simulink model "harnessOpenLoop2"  (R2025b)
settings: Solver=VariableStepAuto  StartTime=0.0  StopTime=600  RelTol=1e-3  AbsTol=1e-3
PreLoadFcn:
  | load DowthermProps.mat
  | load TolueneProps.mat
  | load parameters.mat
undefined symbols (not defined in the file): DOWTHERM_A, NominalStates
libraries: fl_lib x52, nesl_utility x14, SimscapeFluids_lib x6
(part 1 of 2)
settings Model: Creator=ytang  LastModifiedBy=ytang
settings SolverCC: AutoScaleAbsTol=off  AlgebraicLoopSolver=TrustRegion  MaxZcPerStep=1.0
settings DebuggingCC: UnconnectedInputMsg=warning  UnconnectedOutputMsg=warning  UnconnectedLineMsg=warning  SymbolicDimsDataTypeCodeGenerationDiagnostic=none
settings ModelReferenceCC: EnableRefExpFcnMdlSchedulingChecks=on
settings SFSimCC: CustomCodeUndefinedFunction=UseInterfaceOnly
settings RTWCC: GPUComputeCapability=3.5  DLArmComputeVersion=19.05
settings SimscapeCC: SimscapeLogType=all  SimscapeLogSimulationStatistics=on  SimscapeLogDataHistory=10000.0

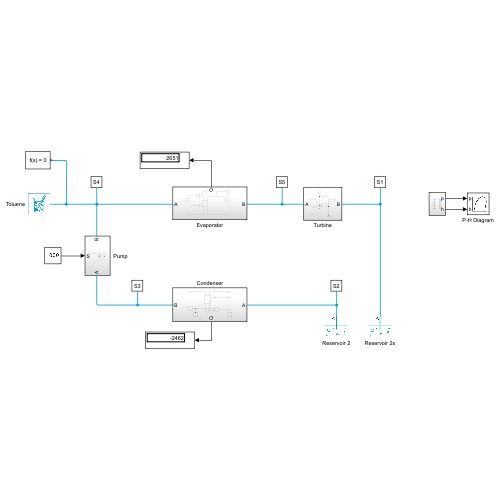
[thumbnail: Simulink's stored preview of the top-level diagram]
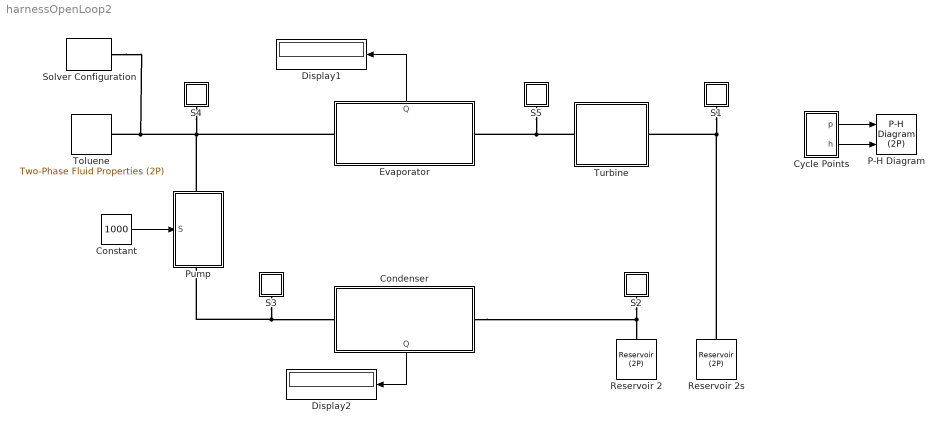
== system harnessOpenLoop2 ==
  Condenser : Subsystem
      settings: PortSchema="{\"entries\":[{\"content\":{\"sides\":[{\"content\":{\"connectorIds\":[\"LConn1\"]},\"type\":\"ConnectorPlacement.EquallySpacedRectSide\",\"uuid\":\"5f0c218a-0034-4896-a5ad-777cf4b77127\"},{\"content\":{\"connectorIds\":[\"RConn1\"],\"side\":\"RIGHT\"},\"type\":\"ConnectorPlacement.EquallySpacedRectSide\",\"uuid\":\"48348978-6e80-4dd2-96bc-6b6e5506de63\"},{\"content\":{\"side\":\"TOP\"},\"type\":\"ConnectorPlacement.EquallySpacedRectSide\",\"uuid\":\"323fdf21-ad06-4626-bb14-e50b2c3800bf\"},{\"content\":{\"connectorIds\":[\"Out1\"],\"side\":\"BOTTOM\"},\"type\":\"ConnectorPlacement.EquallySpacedRectSide\",\"uuid\":\"aca4f6cd-429e-409c-a520-3edf08891ff6\"}]},\"type\":\"ConnectorPlacement.EquallySpacedConnector\",\"uuid\":\"164d264d-504f-434e-a862-7f13511d2ab2\"}],\"packageUris\":[\"http://schema.mathworks.com/mf0/Connector/R2020b\"],\"version\":\"1.0\"}"
  Constant : Constant  Value=1000
  Cycle Points : Subsystem
  Display1 : Display
  Display2 : Display
  Evaporator : Subsystem
      settings: PortSchema="{\"entries\":[{\"content\":{\"sides\":[{\"content\":{\"connectorIds\":[\"LConn1\"]},\"type\":\"ConnectorPlacement.EquallySpacedRectSide\",\"uuid\":\"203ff6bd-d0a3-4ae0-8936-cc55cdbd18f3\"},{\"content\":{\"connectorIds\":[\"RConn1\"],\"side\":\"RIGHT\"},\"type\":\"ConnectorPlacement.EquallySpacedRectSide\",\"uuid\":\"d7ec114f-7f7a-465c-9e8c-44310e9996a8\"},{\"content\":{\"connectorIds\":[\"Out1\"],\"side\":\"TOP\"},\"type\":\"ConnectorPlacement.EquallySpacedRectSide\",\"uuid\":\"8a02f4d6-fd47-469c-93dc-df70d5198f34\"}]},\"type\":\"ConnectorPlacement.EquallySpacedConnector\",\"uuid\":\"0d570563-7e47-4bed-99ef-c8562ff711da\"}],\"packageUris\":[\"http://schema.mathworks.com/mf0/Connector/R2020b\"],\"version\":\"1.0\"}"
  P-H Diagram : SimscapeFluids_lib/Two-Phase Fluid/Utilities/P-H Diagram (2P)  p_unit=MPa  h_unit=kJ/kg
  Pump : Subsystem
      settings: PortSchema="{\"entries\":[{\"content\":{\"sides\":[{\"content\":{\"connectorIds\":[\"In1\"]},\"type\":\"ConnectorPlacement.EquallySpacedRectSide\",\"uuid\":\"bd46a3b8-4e65-4bae-b788-140c87bc05c7\"},{\"content\":{\"side\":\"RIGHT\"},\"type\":\"ConnectorPlacement.EquallySpacedRectSide\",\"uuid\":\"def7fa73-7e7d-4df6-a4d3-5611c09c4867\"},{\"content\":{\"connectorIds\":[\"LConn1\"],\"side\":\"TOP\"},\"type\":\"ConnectorPlacement.EquallySpacedRectSide\",\"uuid\":\"58b0f85b-d673-482e-aa82-3f2e724cb1a3\"},{\"content\":{\"connectorIds\":[\"RConn1\"],\"side\":\"BOTTOM\"},\"type\":\"ConnectorPlacement.EquallySpacedRectSide\",\"uuid\":\"1f6d7ee3-0842-4a9d-bce3-eda34043cffb\"}]},\"type\":\"ConnectorPlacement.EquallySpacedConnector\",\"uuid\":\"d8a4bb42-4f82-479c-8b4b-df8f3b783e33\"}],\"packageUris\":[\"http://schema.mathworks.com/mf0/Connector/R2020b\"],\"version\":\"1.0\"}"
  Reservoir 2 : fl_lib/Two-Phase Fluid/Elements/Reservoir (2P)  pressure_spec=foundation.enum.ReservoirPressureSpec2P.Specified  reservoir_pressure=NominalStates.P(2) MPa  reservoir_condensing_temperature=373.15 K  reservoir_evaporating_temperature=373.15 K  energy_spec=foundation.enum.ReservoirEnergySpec2P.Temperature  reservoir_temperature=NominalStates.T(2) degC  reservoir_quality=0.5  reservoir_void_fraction=0.5  reservoir_enthalpy=1500 kJ/kg  reservoir_internal_energy=1500 kJ/kg  reservoir_subcooling=5 deltaK  reservoir_superheating=5 deltaK  area_A=0.01 m^2
  Reservoir 2s : fl_lib/Two-Phase Fluid/Elements/Reservoir (2P)  pressure_spec=foundation.enum.ReservoirPressureSpec2P.Specified  reservoir_pressure=NominalStates.P(2) MPa  reservoir_condensing_temperature=373.15 K  reservoir_evaporating_temperature=373.15 K  energy_spec=foundation.enum.ReservoirEnergySpec2P.Temperature  reservoir_temperature=NominalStates.T(2) degC  reservoir_quality=0.5  reservoir_void_fraction=0.5  reservoir_enthalpy=1500 kJ/kg  reservoir_internal_energy=1500 kJ/kg  reservoir_subcooling=5 deltaK  reservoir_superheating=5 deltaK  area_A=0.01 m^2
  S1 : Subsystem
      mask Display: disp(get_param(gcb, 'Name'))
  S2 : Subsystem
      mask Display: disp(get_param(gcb, 'Name'))
  S3 : Subsystem
      mask Display: disp(get_param(gcb, 'Name'))
  S4 : Subsystem
      mask Display: disp(get_param(gcb, 'Name'))
  S5 : Subsystem
      mask Display: disp(get_param(gcb, 'Name'))
  Solver Configuration : nesl_utility/Solver Configuration  PhysicalDomain=network_engine_domain  SubClassName=solver  LeftPortType=input  RightPortType=generic  Tones=[]  Harmonics=[]  SimulateNoise=off  Profile=off  UseLocalSampling=off  EnableSwitchedLinearOptims=on  FrequencyDomain=off  UseCCode=off  RelTol=0.001  AbsTol=0.001  MinStep=1e-09  ToWorkspace=off  RevertToSquareIcSolve=off  NumHomotopyIterations=100  PhasorMode=off  PhasorModeNumHarmonics=1  ConsistencySolver=NEWTON_XTOL_AFTER_FTOL  IndexReductionMethod=DerivativeReplacement  DoDC=off  ResidualTolerance=1e-09  ConsistencyTolSource=GLOBAL  ConsistencyAbsTol=0.001  ConsistencyRelTol=0.001  ConsistencyTolFactor=0.001  UseLocalSolver=off  LocalSolverChoice=NE_BACKWARD_EULER_ADVANCER  ResolveIndetEquations=on  FunctionEvalNumThread=1  LocalSolverSampleTime=0.001  DoFixedCost=off  MaxNonlinIter=3  MaxModeIter=2  ComputeImpulses=off  ImpulseIterations=2  LinearAlgebra=auto  LinearAlgebraNumThread=0  EquationFormulation=NE_TIME_EF  DelaysMemoryBudget=1024  AutomaticFiltering=on  FilteringTimeConstant=0.001  PartitionStorageMethod=AS_NEEDED  PartitionMemoryBudget=1024  PartitionMethod=ROBUST  MultibodyUseLocalSolver=off  MultibodyLocalSolverChoice=ODE1  MultibodyLocalSolverSampleTime=0.001
  Toluene : fl_lib/Two-Phase Fluid/Utilities/Two-Phase Fluid Properties (2P)  u_min=Toluene.u_min kJ/kg  u_max=Toluene.u_max kJ/kg  p_TLU=Toluene.p MPa  p_crit=Toluene.p_crit MPa  critical_region=foundation.enum.critical_region.clip  p_crit_fraction=0.12  p_atm=0.101325 MPa  properties_range_check=simscape.enum.assert.action.error  q_rev=0.01 Pa  unorm_liq=Toluene.liquid.unorm  v_liq=Toluene.liquid.v m^3/kg  s_liq=Toluene.liquid.s kJ/(kg*K)  T_liq=Toluene.liquid.T K  nu_liq=Toluene.liquid.nu mm^2/s  k_liq=Toluene.liquid.k W/(m*K)  Pr_liq=Toluene.liquid.Pr  u_sat_liq=Toluene.liquid.u_sat kJ/kg  unorm_vap=Toluene.vapor.unorm  v_vap=Toluene.vapor.v m^3/kg  s_vap=Toluene.vapor.s kJ/(kg*K)  T_vap=Toluene.vapor.T K  nu_vap=Toluene.vapor.nu mm^2/s  k_vap=Toluene.vapor.k W/(m*K)  Pr_vap=Toluene.vapor.Pr  u_sat_vap=Toluene.vapor.u_sat kJ/kg
      settings: InternalSimscapePortConfiguration="{\"Bottom\":[],\"Left\":[],\"Right\":[{\"id\":\"A\",\"label\":\"\",\"type\":\"foundation.two_phase_fluid.two_phase_fluid\"}],\"Top\":[]}"
  Turbine : Subsystem
  wires:
  Cycle Points/2(h) -> P-H Diagram/2
  Cycle Points/1(p) -> P-H Diagram/1
  Constant/1 -> Pump/1(S)
  Evaporator/1(Q) -> Display1/1
  Condenser/1(Q) -> Display2/1
  connections:
  Turbine/LConn1 -- S5/LConn1 -- Evaporator/RConn1
  S2/LConn1 -- Condenser/RConn1 -- Reservoir 2/LConn1
  S3/LConn1 -- Pump/RConn1 -- Condenser/LConn1
  Pump/LConn1 -- S4/LConn1 -- Evaporator/LConn1 -- Solver Configuration/RConn1 -- Toluene/RConn1
  Reservoir 2s/LConn1 -- S1/LConn1 -- Turbine/RConn1

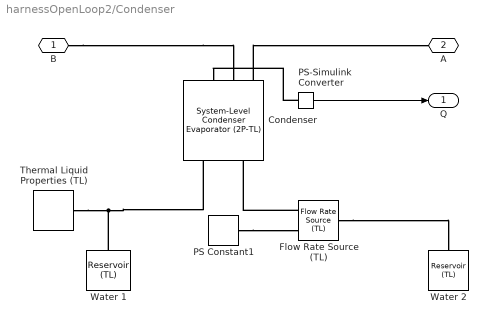
== system harnessOpenLoop2/Condenser ==
  Condenser : SimscapeFluids_lib/Heat Exchangers/Two-Phase Fluid - Thermal Liquid/System-Level Condenser Evaporator (2P-TL)  flow_arrangement=fluids.heat_exchangers.enum.SystemLevelFlowArrangement2PTL.Counter  wall_thermal_mass=false  mass_wall=1 kg  cp_wall=490 J/(K*kg)  nominal_init_wall=true  T_wall_init=293.15 K  area_A1=0.01 m^2  area_B1=0.01 m^2  area_A2=0.01 m^2  area_B2=0.01 m^2  operating_condition_2P=fluids.heat_exchangers.enum.SystemLevelOperatingCondition2PTL.Condenser  mdot_nominal_2P=Condenser.Fluid.mdot kg/s  delta_p_nominal_2P=0.0001 MPa  pressure_spec_cond_2P=fluids.heat_exchangers.enum.SystemLevelPressureSpecCondenser2P.InletPressure  pressure_spec_evap_2P=fluids.heat_exchangers.enum.SystemLevelPressureSpecEvaporator2P.InletPressure  p_in_nominal_2P=NominalStates.P(2) MPa  T_cond_nominal_2P=313.15 K  T_evap_nominal_2P=243.15 K  inlet_spec_2P=fluids.heat_exchangers.enum.SystemLevelInletSpec2P.Temperature  T_in_nominal_2P=NominalStates.T(2) degC  h_in_nominal_2P=440 kJ/kg  x_in_nominal_2P=1  capacity_spec_2P=fluids.heat_exchangers.enum.SystemLevelCapacitySpec.HeatTransfer  Q_nominal=Condenser.Heat kW  outlet_spec_cond_2P=fluids.heat_exchangers.enum.SystemLevelOutletSpecCondenser2P.Enthalpy  outlet_spec_evap_2P=fluids.heat_exchangers.enum.SystemLevelOutletSpecEvaporator2P.Enthalpy  delta_T_sub_nominal_2P=5 deltaK  delta_T_sup_nominal_2P=5 deltaK  h_out_nominal_2P=250 kJ/kg  x_out_nominal_2P=0  volume_2P=0.2 m^3  nominal_init_2P=true  energy_spec_2P=foundation.enum.energy_spec.enthalpy  p_init_2P=0.101325 MPa  T_init_2P=293.15 K  x_init_2P=0.5  alpha_init_2P=0.5  h_init_2P=1500 kJ/kg  u_init_2P=1500 kJ/kg  mdot_nominal_TL=Condenser.Water.mdot kg/s  delta_p_nominal_TL=0.0001 MPa  p_in_nominal_TL=0.101325 MPa  T_in_nominal_TL=Condenser.Water.Tin degC  volume_TL=0.2 m^3  nominal_init_TL=true  p_init_TL=0.101325 MPa  T_init_TL=293.15 K  a_liq_2P=0.023  a_mix_2P=0.005  a_vap_2P=0.023  b_2P=0.8  c_2P=0.33  a_TL=0.023  b_TL=0.8  c_TL=0.33
      settings: InternalSimscapePortConfiguration="{\"Bottom\":[],\"Left\":[{\"id\":\"A1\",\"label\":\"A1\",\"type\":\"foundation.two_phase_fluid.two_phase_fluid\"},{\"id\":\"B1\",\"label\":\"B1\",\"type\":\"foundation.two_phase_fluid.two_phase_fluid\"}],\"Right\":[{\"id\":\"A2\",\"label\":\"A2\",\"type\":\"foundation.thermal_liquid.thermal_liquid\"},{\"id\":\"B2\",\"label\":\"B2\",\"type\":\"foundation.thermal_liquid.thermal_liquid\"}],\"Top\":[{\"id\":\"Q1\",\"label\":\"Q1\",\"type\":\"output\"},{\"id\":\"Q2\",\"label\":\"Q2\",\"type\":\"output\"}]}"
  Flow Rate Source (TL) : fl_lib/Thermal Liquid/Sources/Flow Rate Source (TL)  source_type=foundation.enum.constant_controlled.controlled  flow_type=foundation.enum.mass_volumetric_flow.mass  mass_flow=0 kg/s  volumetric_flow=0 m^3/s  power_spec=foundation.enum.power_spec.isentropic  area=0.01 m^2
  PS Constant1 : fl_lib/Physical Signals/Sources/PS Constant  constant=Condenser.Water.mdot kg/s
  PS-Simulink Converter : nesl_utility/PS-Simulink Converter  PhysicalDomain=network_engine_domain  SubClassName=ps_output  LeftPortType=input  RightPortType=output  PseudoPeriodic=off  Frequencies=[]  VectorFormat=inherit  Unit=kW  AffineConversion=off
  Thermal Liquid Properties (TL) : SimscapeFluids_lib/Thermal Liquid/Utilities/Thermal Liquid Properties (TL)  fluid_list=fluids.thermal_liquid.utilities.enum.thermal_liquid_fluid_list.water  concentration_param_EG=fluids.thermal_liquid.utilities.enum.thermal_liquid_concentration.volume_fraction  concentration_param_PG=fluids.thermal_liquid.utilities.enum.thermal_liquid_concentration.volume_fraction  c_mass_SW=3.5e-3  c_mass_EG=0.1  c_mass_PG=0.1  c_mass_GL=0.1  c_vol_EG=0.1  c_vol_PG=0.1  beta_const_EG=2.1791 GPa  beta_const_PG=2.1791 GPa  beta_const_GL=2.1791 GPa  p_min_EG=0.01 MPa  p_min_PG=0.01 MPa  p_min_GL=0.01 MPa  p_max_EG=50 MPa  p_max_PG=50 MPa  p_max_GL=50 MPa  p_atm=0.101325 MPa  properties_range_check=simscape.enum.assert.action.error
  Water 1 : fl_lib/Thermal Liquid/Elements/Reservoir (TL)  pressure_spec=foundation.enum.pressure_spec.atmospheric  reservoir_pressure=0.101325 MPa  reservoir_temperature=Condenser.Water.Tin degC  area=0.01 m^2
  Water 2 : fl_lib/Thermal Liquid/Elements/Reservoir (TL)  pressure_spec=foundation.enum.pressure_spec.atmospheric  reservoir_pressure=0.101325 MPa  reservoir_temperature=Condenser.Water.Tout degC  area=0.01 m^2
  B : PMIOPort  Side=Left
  A : PMIOPort  Port=2  Side=Right
  Q : Outport
  wires:
  PS-Simulink Converter/1 -> Q/1
  connections:
  Flow Rate Source (TL)/RConn1 -- Water 2/LConn1
  PS-Simulink Converter/LConn1 -- Condenser/LConn3
  Water 1/LConn1 -- Condenser/RConn2 -- Thermal Liquid Properties (TL)/RConn1
  Flow Rate Source (TL)/LConn1 -- Condenser/RConn1
  PS Constant1/RConn1 -- Flow Rate Source (TL)/LConn2
  B/RConn1 -- Condenser/LConn2
  Condenser/LConn1 -- A/RConn1

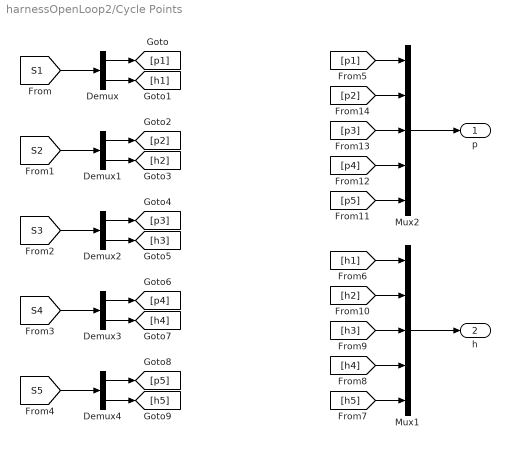
== system harnessOpenLoop2/Cycle Points ==
  Demux{,1..4} (5 alike) : Demux  Outputs=2
  Mux1 : Mux  Inputs=5
  Mux2 : Mux  Inputs=5
  p : Outport
  h : Outport  Port=2
  wires:
  Mux1/1 -> h/1
  [S1] -> Demux/1
  [S2] -> Demux1/1
  [S3] -> Demux2/1
  [S4] -> Demux3/1
  [S5] -> Demux4/1
  Mux2/1 -> p/1
  Demux/1 -> [p1]
  [p1] -> Mux2/1
  Demux2/2 -> [h3]
  [h3] -> Mux1/3
  Demux3/2 -> [h4]
  [h4] -> Mux1/4
  Demux4/2 -> [h5]
  [h5] -> Mux1/5
  Demux1/2 -> [h2]
  [h2] -> Mux1/2
  Demux/2 -> [h1]
  [h1] -> Mux1/1
  Demux3/1 -> [p4]
  [p4] -> Mux2/4
  Demux4/1 -> [p5]
  [p5] -> Mux2/5
  Demux1/1 -> [p2]
  [p2] -> Mux2/2
  Demux2/1 -> [p3]
  [p3] -> Mux2/3

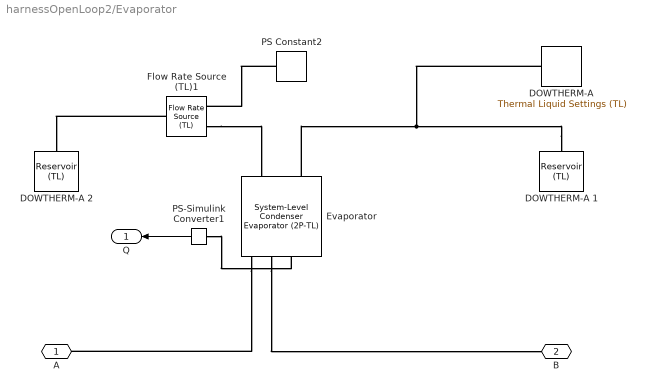
== system harnessOpenLoop2/Evaporator ==
  DOWTHERM-A : fl_lib/Thermal Liquid/Utilities/Thermal Liquid Settings (TL)  table_dimensions=foundation.enum.table_dimensions_TL.one_dimensional  T_TLU=DOWTHERM_A.T degC  p_TLU=[0.01, 0.1, 5 : 5 : 50] MPa  p_atm=0.101325 MPa  pT_region_flag=foundation.enum.pT_region_TL.min_max  T_min=273.16 K  T_max=373.16 K  p_min=0.01 MPa  p_max=50 MPa  T_min_1D=DOWTHERM_A.T(1) degC  T_max_1D=DOWTHERM_A.T(end) degC  p_min_1D=0.01 MPa  p_max_1D=50 MPa  pT_validity_TLU=[1, 1, 1, 1, 1, 1, 1, 1, 1, 1, 1, 1; 1, 1, 1, 1, 1, 1, 1, 1, 1, 1, 1, 1; 1, 1, 1, 1, 1, 1, 1, 1, 1, 1, 1, 1; 1, 1, 1, 1, 1, 1, 1, 1, 1, 1, 1, 1; 1, 1, 1, 1, 1, 1, 1, 1, 1, 1, 1, 1; 0, 1, 1, 1, 1, 1, 1, 1, 1, 1, 1, 1; 0, 1, 1, 1, 1, 1, 1, 1, 1, 1, 1, 1; 0, 1, 1, 1, 1, 1, 1, 1, 1, 1, 1, 1; 0, 1, 1, 1, 1, 1, 1, 1, 1, 1, 1, 1; 0, 1, 1, 1, 1, 1, 1, 1, 1, 1, 1, 1; 0, 0, 1, 1, 1, 1, 1, 1, 1, 1, 1, 1]  properties_range_check=simscape.enum.assert.action.error  rho_parameterization_2D=foundation.enum.rho_parameterization_2D.rho_beta_alpha  rho_parameterization_1D=foundation.enum.rho_parameterization_1D.rho_vector  rho_TLU=[999.7973, 999.8431, 1002.3216, 1004.8218, 1007.293, 1009.7358, 1012.1506, 1014.5379, 1016.8979, 1019.2311, 1021.538, 1023.8188; 999.6579, 999.7009, 1002.0303, 1004.382, 1006.7084, 1009.0101, 1011.2874, 1013.5407, 1015.7703, 1017.9766, 1020.1599, 1022.3206; 998.1632, 998.2045, 1000.4375, 1002.6924, 1004.9239, 1007.1324, 1009.3183, 1011.4819, 1013.6236, 1015.7438, 1017.8428, 1019.921; 995.6057, 995.6458, 997.8186, 1000.0128, 1002.1841, 1004.3332, 1006.4603, 1008.566, 1010.6505, 1012.7144, 1014.758, 1016.7815; 992.1724, 992.2119, 994.3513, 996.5113, 998.6484, 1000.7633, 1002.8563, 1004.928, 1006.9788, 1009.009, 1011.0192, 1013.0097; 988.02, 988.0299, 990.1568, 992.3035, 994.4268, 996.5273, 998.6056, 1000.6622, 1002.6976, 1004.7123, 1006.7067, 1008.6813; 983.18, 983.1901, 985.3217, 987.4721, 989.5983, 991.7008, 993.7803, 995.8374, 997.8726, 999.8864, 1001.8795, 1003.8522; 977.75, 977.7583, 979.9094, 982.0783, 984.2216, 986.34, 988.4343, 990.505, 992.5529, 994.5786, 996.5825, 998.5654; 971.77, 971.7836, 973.9673, 976.1678, 978.3409, 980.4876, 982.6087, 984.7049, 986.7768, 988.8254, 990.8511, 992.8545; 965.26, 965.3023, 967.5311, 969.7753, 971.9901, 974.1764, 976.3354, 978.4676, 980.5741, 982.6556, 984.7129, 986.7465; 958.62, 958.6315, 960.627, 962.9267, 965.1944, 967.4314, 969.6387, 971.8173, 973.9681, 976.0921, 978.19, 980.2628] kg/m^3  beta_TLU=[1.9649, 1.9654, 1.9929, 2.0213, 2.0499, 2.0787, 2.1078, 2.1372, 2.1668, 2.1966, 2.2268, 2.2572; 2.0913, 2.0918, 2.1191, 2.1471, 2.1752, 2.2036, 2.2322, 2.261, 2.2899, 2.3191, 2.3485, 2.3781; 2.1786, 2.1791, 2.2067, 2.235, 2.2634, 2.2919, 2.3206, 2.3494, 2.3784, 2.4075, 2.4367, 2.4661; 2.2332, 2.2337, 2.2619, 2.2908, 2.3197, 2.3487, 2.3778, 2.407, 2.4363, 2.4657, 2.4951, 2.5246; 2.26, 2.2605, 2.2895, 2.3191, 2.3487, 2.3784, 2.4081, 2.4378, 2.4675, 2.4973, 2.5272, 2.5571; 2.2638, 2.2638, 2.2936, 2.324, 2.3544, 2.3848, 2.4151, 2.4455, 2.4758, 2.5062, 2.5365, 2.5669; 2.2472, 2.2472, 2.2779, 2.3092, 2.3403, 2.3715, 2.4025, 2.4336, 2.4646, 2.4955, 2.5264, 2.5573; 2.214, 2.214, 2.2455, 2.2776, 2.3096, 2.3415, 2.3733, 2.405, 2.4367, 2.4683, 2.4998, 2.5313; 2.1668, 2.1668, 2.1992, 2.2321, 2.2649, 2.2976, 2.3301, 2.3626, 2.3949, 2.4272, 2.4593, 2.4914; 2.1081, 2.1081, 2.1413, 2.175, 2.2086, 2.2421, 2.2754, 2.3085, 2.3415, 2.3744, 2.4072, 2.4399; 2.0494, 2.0494, 2.0739, 2.1084, 2.1428, 2.177, 2.211, 2.2449, 2.2786, 2.3121, 2.3455, 2.3788] GPa  alpha_TLU=1e-4 * [-.679, -.676, -.49, -.307, -.13, .041, .206, .365, .519, .668, .811, .949; .878, .881, .998, 1.114, 1.227, 1.337, 1.445, 1.549, 1.651, 1.75, 1.846, 1.939; 2.068, 2.069, 2.141, 2.213, 2.283, 2.352, 2.42, 2.486, 2.551, 2.614, 2.676, 2.736; 3.034, 3.035, 3.074, 3.113, 3.152, 3.191, 3.229, 3.267, 3.305, 3.341, 3.377, 3.413; 3.855, 3.856, 3.87, 3.884, 3.899, 3.914, 3.93, 3.946, 3.961, 3.977, 3.993, 4.009; 4.578, 4.578, 4.572, 4.566, 4.562, 4.558, 4.555, 4.552, 4.55, 4.549, 4.548, 4.547; 5.233, 5.233, 5.209, 5.186, 5.165, 5.144, 5.125, 5.107, 5.09, 5.074, 5.059, 5.045; 5.84, 5.84, 5.801, 5.762, 5.725, 5.691, 5.657, 5.625, 5.595, 5.566, 5.538, 5.512; 6.414, 6.414, 6.36, 6.307, 6.256, 6.208, 6.161, 6.117, 6.074, 6.033, 5.994, 5.956; 6.967, 6.967, 6.898, 6.831, 6.766, 6.705, 6.646, 6.589, 6.535, 6.482, 6.432, 6.384; 7.519, 7.519, 7.423, 7.342, 7.264, 7.189, 7.118, 7.049, 6.983, 6.92, 6.859, 6.8] 1/K  rho_TLU_2=[999.7973, 999.8431, 1002.3216, 1004.8218, 1007.293, 1009.7358, 1012.1506, 1014.5379, 1016.8979, 1019.2311, 1021.538, 1023.8188; 999.6579, 999.7009, 1002.0303, 1004.382, 1006.7084, 1009.0101, 1011.2874, 1013.5407, 1015.7703, 1017.9766, 1020.1599, 1022.3206; 998.1632, 998.2045, 1000.4375, 1002.6924, 1004.9239, 1007.1324, 1009.3183, 1011.4819, 1013.6236, 1015.7438, 1017.8428, 1019.921; 995.6057, 995.6458, 997.81864, 1000.0128, 1002.1841, 1004.3332, 1006.4603, 1008.566, 1010.6505, 1012.7144, 1014.758, 1016.7815; 992.1724, 992.2119, 994.3513, 996.5113, 998.6484, 1000.7633, 1002.8563, 1004.928, 1006.9788, 1009.009, 1011.0192, 1013.0097; 988.02, 988.0299, 990.1568, 992.3035, 994.4268, 996.5273, 998.6056, 1000.6622, 1002.6976, 1004.7123, 1006.7067, 1008.6813; 983.18, 983.1901, 985.3217, 987.4721, 989.5983, 991.7008, 993.7803, 995.8374, 997.8726, 999.8864, 1001.8795, 1003.8522; 977.75, 977.7583, 979.9094, 982.0783, 984.2216, 986.34, 988.4343, 990.505, 992.5529, 994.5786, 996.5825, 998.5654; 971.77, 971.7836, 973.9673, 976.1678, 978.3409, 980.4876, 982.6087, 984.7049, 986.7768, 988.8254, 990.8511, 992.8545; 965.26, 965.3023, 967.5311, 969.7753, 971.9901, 974.1764, 976.3354, 978.4676, 980.5741, 982.6556, 984.7129, 986.7465; 958.62, 958.6315, 960.627, 962.9267, 965.1944, 967.4314, 969.6387, 971.8173, 973.9681, 976.0921, 978.19, 980.2628] kg/m^3  rho_ref_3=998.21 kg/m^3  T_ref_3=293.16 K  p_ref_3=0.101325 MPa  beta_const_3=2.1791 GPa  alpha_const_3=2.0691e-4 1/K  rho_TLU_4=DOWTHERM_A.rho kg/m^3  beta_const_4=0.5 GPa  p_ref_4=0.101325 MPa  rho_ref_5=998.21 kg/m^3  T_ref_5=293.16 K  p_ref_5=0.101325 MPa  beta_const_5=2.1791 GPa  alpha_const_5=2.0691e-4 1/K  u_parameterization_2D=foundation.enum.u_parameterization_2D.u_cp  u_parameterization_1D=foundation.enum.u_parameterization_1D.cp  u_TLU=[.0002, .0018, .086, .1588, .219, .267, .3034, .3288, .3436, .3483, .3435, .3294; 42.062, 42.06, 41.935, 41.804, 41.668, 41.527, 41.382, 41.233, 41.081, 40.924, 40.763, 40.599; 83.953, 83.948, 83.651, 83.349, 83.049, 82.749, 82.451, 82.153, 81.856, 81.56, 81.265, 80.971; 125.77, 125.76, 125.31, 124.86, 124.41, 123.97, 123.53, 123.1, 122.68, 122.25, 121.84, 121.42; 167.57, 167.56, 166.96, 166.37, 165.79, 165.21, 164.65, 164.09, 163.54, 163, 162.46, 161.94; 209.36, 209.36, 208.63, 207.9, 207.19, 206.48, 205.79, 205.11, 204.45, 203.79, 203.14, 202.5; 251.19, 251.19, 250.33, 249.47, 248.62, 247.79, 246.98, 246.18, 245.39, 244.62, 243.86, 243.12; 293.06, 293.06, 292.07, 291.07, 290.1, 289.14, 288.2, 287.28, 286.38, 285.49, 284.62, 283.77; 334.99, 334.99, 333.86, 332.73, 331.63, 330.54, 329.48, 328.44, 327.41, 326.41, 325.43, 324.46; 377, 377, 375.73, 374.46, 373.22, 372, 370.81, 369.64, 368.5, 367.38, 366.27, 365.19; 419.01, 419.01, 417.69, 416.27, 414.89, 413.54, 412.21, 410.91, 409.64, 408.4, 407.17, 405.98] kJ/kg  cp_TLU=[4.2199, 4.2194, 4.1957, 4.1726, 4.1508, 4.13, 4.1103, 4.0916, 4.0738, 4.0569, 4.0408, 4.0254; 4.1955, 4.1951, 4.1769, 4.1592, 4.1422, 4.1259, 4.1103, 4.0954, 4.0812, 4.0676, 4.0545, 4.0421; 4.1843, 4.184, 4.169, 4.1543, 4.1401, 4.1264, 4.1133, 4.1007, 4.0885, 4.0768, 4.0656, 4.0548; 4.1801, 4.1798, 4.1667, 4.1538, 4.1413, 4.1293, 4.1177, 4.1064, 4.0956, 4.0851, 4.075, 4.0653; 4.1796, 4.1794, 4.1675, 4.1558, 4.1444, 4.1334, 4.1227, 4.1123, 4.1023, 4.0926, 4.0832, 4.0741; 4.1813, 4.1813, 4.1702, 4.1592, 4.1484, 4.138, 4.1279, 4.1181, 4.1086, 4.0993, 4.0903, 4.0816; 4.185, 4.185, 4.1742, 4.1636, 4.1532, 4.1432, 4.1334, 4.1239, 4.1146, 4.1056, 4.0969, 4.0884; 4.1901, 4.1901, 4.1795, 4.169, 4.1588, 4.1489, 4.1393, 4.1299, 4.1207, 4.1118, 4.1032, 4.0947; 4.1968, 4.1968, 4.1862, 4.1757, 4.1655, 4.1555, 4.1458, 4.1364, 4.1273, 4.1183, 4.1096, 4.1012; 4.2052, 4.2052, 4.1944, 4.1837, 4.1733, 4.1632, 4.1534, 4.1438, 4.1345, 4.1255, 4.1166, 4.108; 4.2136, 4.2136, 4.2045, 4.1935, 4.1828, 4.1724, 4.1623, 4.1524, 4.1429, 4.1335, 4.1245, 4.1157] kJ/(K*kg)  u_TLU_2=[.0002, .0018, .086, .1588, .219, .267, .3034, .3288, .3436, .3483, .3435, .3294; 42.062, 42.06, 41.935, 41.804, 41.668, 41.527, 41.382, 41.233, 41.081, 40.924, 40.763, 40.599; 83.953, 83.948, 83.651, 83.349, 83.049, 82.749, 82.451, 82.153, 81.856, 81.56, 81.265, 80.971; 125.77, 125.76, 125.31, 124.86, 124.41, 123.97, 123.53, 123.1, 122.68, 122.25, 121.84, 121.42; 167.57, 167.56, 166.96, 166.37, 165.79, 165.21, 164.65, 164.09, 163.54, 163, 162.46, 161.94; 209.36, 209.36, 208.63, 207.9, 207.19, 206.48, 205.79, 205.11, 204.45, 203.79, 203.14, 202.5; 251.19, 251.19, 250.33, 249.47, 248.62, 247.79, 246.98, 246.18, 245.39, 244.62, 243.86, 243.12; 293.06, 293.06, 292.07, 291.07, 290.1, 289.14, 288.2, 287.28, 286.38, 285.49, 284.62, 283.77; 334.99, 334.99, 333.86, 332.73, 331.63, 330.54, 329.48, 328.44, 327.41, 326.41, 325.43, 324.46; 377, 377, 375.73, 374.46, 373.22, 372, 370.81, 369.64, 368.5, 367.38, 366.27, 365.19; 419.01, 419.01, 417.69, 416.27, 414.89, 413.54, 412.21, 410.91, 409.64, 408.4, 407.17, 405.98] kJ/kg  cp_TLU_3=[4.2199, 4.2194, 4.1957, 4.1726, 4.1508, 4.13, 4.1103, 4.0916, 4.0738, 4.0569, 4.0408, 4.0254; 4.1955, 4.1951, 4.1769, 4.1592, 4.1422, 4.1259, 4.1103, 4.0954, 4.0812, 4.0676, 4.0545, 4.0421; 4.1843, 4.184, 4.169, 4.1543, 4.1401, 4.1264, 4.1133, 4.1007, 4.0885, 4.0768, 4.0656, 4.0548; 4.1801, 4.1798, 4.1667, 4.1538, 4.1413, 4.1293, 4.1177, 4.1064, 4.0956, 4.0851, 4.075, 4.0653; 4.1796, 4.1794, 4.1675, 4.1558, 4.1444, 4.1334, 4.1227, 4.1123, 4.1023, 4.0926, 4.0832, 4.0741; 4.1813, 4.1813, 4.1702, 4.1592, 4.1484, 4.138, 4.1279, 4.1181, 4.1086, 4.0993, 4.0903, 4.0816; 4.185, 4.185, 4.1742, 4.1636, 4.1532, 4.1432, 4.1334, 4.1239, 4.1146, 4.1056, 4.0969, 4.0884; 4.1901, 4.1901, 4.1795, 4.169, 4.1588, 4.1489, 4.1393, 4.1299, 4.1207, 4.1118, 4.1032, 4.0947; 4.1968, 4.1968, 4.1862, 4.1757, 4.1655, 4.1555, 4.1458, 4.1364, 4.1273, 4.1183, 4.1096, 4.1012; 4.2052, 4.2052, 4.1944, 4.1837, 4.1733, 4.1632, 4.1534, 4.1438, 4.1345, 4.1255, 4.1166, 4.108; 4.2136, 4.2136, 4.2045, 4.1935, 4.1828, 4.1724, 4.1623, 4.1524, 4.1429, 4.1335, 4.1245, 4.1157] kJ/(K*kg)  u_TLU_4=[.0018; 42.06; 83.948; 125.76; 167.56; 209.36; 251.19; 293.06; 334.99; 377; 418.01] kJ/kg  cp_TLU_5=DOWTHERM_A.Cp kJ/(K*kg)  nu_TLU=[1.7917, 1.7914, 1.7763, 1.7615, 1.7473, 1.7338, 1.7208, 1.7085, 1.6967, 1.6854, 1.6747, 1.6645; 1.3061, 1.3059, 1.2986, 1.2914, 1.2845, 1.2779, 1.2716, 1.2656, 1.2598, 1.2543, 1.2491, 1.2441; 1.0032, 1.0032, .9995, .9959, .9924, .9891, .9859, .9829, .9801, .9774, .9748, .9724; .8006, .8005, .7987, .797, .7953, .7937, .7922, .7908, .7894, .7881, .787, .7859; .6577, .6577, .657, .6562, .6555, .6548, .6543, .6537, .6532, .6528, .6523, .652; .553, .553, .5529, .5527, .5526, .5525, .5524, .5524, .5524, .5524, .5524, .5525; .4739, .4739, .4741, .4743, .4745, .4747, .475, .4753, .4755, .4758, .4762, .4765; .4127, .4127, .4131, .4135, .4139, .4143, .4148, .4152, .4157, .4162, .4167, .4172; .3643, .3643, .3648, .3654, .3659, .3665, .367, .3676, .3682, .3688, .3694, .37; .3254, .3254, .3261, .3267, .3273, .328, .3286, .3293, .3299, .3306, .3312, .3319; .2866, .2866, .2945, .2952, .2959, .2965, .2972, .2979, .2986, .2993, .3, .3007] mm^2/s  nu_TLU_2=DOWTHERM_A.nu m^2/s  k_TLU=[561.04, 561.09, 563.8, 566.56, 569.32, 572.08, 574.82, 577.54, 580.24, 582.92, 585.57, 588.18; 580.02, 580.07, 582.45, 584.88, 587.32, 589.75, 592.18, 594.61, 597.02, 599.42, 601.8, 604.16; 598.44, 598.48, 600.73, 603.03, 605.33, 607.64, 609.94, 612.24, 614.54, 616.82, 619.1, 621.36; 615.48, 615.52, 617.73, 620, 622.26, 624.54, 626.81, 629.07, 631.34, 633.6, 635.85, 638.09; 630.6, 630.64, 632.87, 635.15, 637.44, 639.72, 642.01, 644.29, 646.57, 648.84, 651.11, 653.36; 643.61, 643.61, 645.88, 648.21, 650.53, 652.86, 655.18, 657.51, 659.82, 662.14, 664.44, 666.74; 654.39, 654.39, 656.73, 659.12, 661.5, 663.89, 666.27, 668.65, 671.02, 673.38, 675.74, 678.09; 663.13, 663.13, 665.54, 668, 670.46, 672.91, 675.36, 677.8, 680.24, 682.67, 685.09, 687.5; 670.02, 670.02, 672.51, 675.05, 677.59, 680.12, 682.64, 685.16, 687.67, 690.17, 692.66, 695.14; 675.27, 675.27, 677.85, 680.48, 683.11, 685.73, 688.34, 690.94, 693.53, 696.11, 698.68, 701.24; 680.52, 680.52, 681.77, 684.5, 687.22, 689.94, 692.64, 695.34, 698.02, 700.69, 703.35, 706] mW/(K*m)  k_TLU_2=DOWTHERM_A.k W/(K*m)
  DOWTHERM-A 1 : fl_lib/Thermal Liquid/Elements/Reservoir (TL)  pressure_spec=foundation.enum.pressure_spec.atmospheric  reservoir_pressure=0.101325 MPa  reservoir_temperature=Evaporator.Oil.Tin degC  area=0.01 m^2
  DOWTHERM-A 2 : fl_lib/Thermal Liquid/Elements/Reservoir (TL)  pressure_spec=foundation.enum.pressure_spec.atmospheric  reservoir_pressure=0.101325 MPa  reservoir_temperature=Evaporator.Oil.Tout degC  area=0.01 m^2
  Evaporator : SimscapeFluids_lib/Heat Exchangers/Two-Phase Fluid - Thermal Liquid/System-Level Condenser Evaporator (2P-TL)  flow_arrangement=fluids.heat_exchangers.enum.SystemLevelFlowArrangement2PTL.Counter  wall_thermal_mass=false  mass_wall=1 kg  cp_wall=490 J/(K*kg)  nominal_init_wall=true  T_wall_init=293.15 K  area_A1=0.01 m^2  area_B1=0.01 m^2  area_A2=0.01 m^2  area_B2=0.01 m^2  operating_condition_2P=fluids.heat_exchangers.enum.SystemLevelOperatingCondition2PTL.Evaporator  mdot_nominal_2P=Evaporator.Fluid.mdot kg/s  delta_p_nominal_2P=0.0001 MPa  pressure_spec_cond_2P=fluids.heat_exchangers.enum.SystemLevelPressureSpecCondenser2P.InletPressure  pressure_spec_evap_2P=fluids.heat_exchangers.enum.SystemLevelPressureSpecEvaporator2P.InletPressure  p_in_nominal_2P=NominalStates.P(4) MPa  T_cond_nominal_2P=313.15 K  T_evap_nominal_2P=243.15 K  inlet_spec_2P=fluids.heat_exchangers.enum.SystemLevelInletSpec2P.Temperature  T_in_nominal_2P=NominalStates.T(4) degC  h_in_nominal_2P=440 kJ/kg  x_in_nominal_2P=1  capacity_spec_2P=fluids.heat_exchangers.enum.SystemLevelCapacitySpec.HeatTransfer  Q_nominal=Evaporator.Heat kW  outlet_spec_cond_2P=fluids.heat_exchangers.enum.SystemLevelOutletSpecCondenser2P.Enthalpy  outlet_spec_evap_2P=fluids.heat_exchangers.enum.SystemLevelOutletSpecEvaporator2P.Enthalpy  delta_T_sub_nominal_2P=5 deltaK  delta_T_sup_nominal_2P=5 deltaK  h_out_nominal_2P=250 kJ/kg  x_out_nominal_2P=0  volume_2P=0.2 m^3  nominal_init_2P=true  energy_spec_2P=foundation.enum.energy_spec.enthalpy  p_init_2P=0.101325 MPa  T_init_2P=293.15 K  x_init_2P=0.5  alpha_init_2P=0.5  h_init_2P=1500 kJ/kg  u_init_2P=1500 kJ/kg  mdot_nominal_TL=Evaporator.Oil.mdot kg/s  delta_p_nominal_TL=0.0001 MPa  p_in_nominal_TL=0.101325 MPa  T_in_nominal_TL=Evaporator.Oil.Tin degC  volume_TL=0.2 m^3  nominal_init_TL=true  p_init_TL=0.101325 MPa  T_init_TL=293.15 K  a_liq_2P=0.023  a_mix_2P=0.005  a_vap_2P=0.023  b_2P=0.8  c_2P=0.33  a_TL=0.023  b_TL=0.8  c_TL=0.33
      settings: InternalSimscapePortConfiguration="{\"Bottom\":[],\"Left\":[{\"id\":\"A1\",\"label\":\"A1\",\"type\":\"foundation.two_phase_fluid.two_phase_fluid\"},{\"id\":\"B1\",\"label\":\"B1\",\"type\":\"foundation.two_phase_fluid.two_phase_fluid\"}],\"Right\":[{\"id\":\"A2\",\"label\":\"A2\",\"type\":\"foundation.thermal_liquid.thermal_liquid\"},{\"id\":\"B2\",\"label\":\"B2\",\"type\":\"foundation.thermal_liquid.thermal_liquid\"}],\"Top\":[{\"id\":\"Q1\",\"label\":\"Q1\",\"type\":\"output\"},{\"id\":\"Q2\",\"label\":\"Q2\",\"type\":\"output\"}]}"
  Flow Rate Source (TL)1 : fl_lib/Thermal Liquid/Sources/Flow Rate Source (TL)  source_type=foundation.enum.constant_controlled.controlled  flow_type=foundation.enum.mass_volumetric_flow.mass  mass_flow=0 kg/s  volumetric_flow=0 m^3/s  power_spec=foundation.enum.power_spec.isentropic  area=0.01 m^2
  PS Constant2 : fl_lib/Physical Signals/Sources/PS Constant  constant=Evaporator.Oil.mdot kg/s
  PS-Simulink Converter1 : nesl_utility/PS-Simulink Converter  PhysicalDomain=network_engine_domain  SubClassName=ps_output  LeftPortType=input  RightPortType=output  PseudoPeriodic=off  Frequencies=[]  VectorFormat=inherit  Unit=kW  AffineConversion=off
  A : PMIOPort  Side=Left
  B : PMIOPort  Port=2  Side=Right
  Q : Outport
  wires:
  PS-Simulink Converter1/1 -> Q/1
  connections:
  DOWTHERM-A 1/LConn1 -- DOWTHERM-A/RConn1 -- Evaporator/RConn2
  Evaporator/LConn2 -- B/RConn1
  Evaporator/LConn1 -- A/RConn1
  PS Constant2/RConn1 -- Flow Rate Source (TL)1/LConn2
  Flow Rate Source (TL)1/LConn1 -- Evaporator/RConn1
  PS-Simulink Converter1/LConn1 -- Evaporator/LConn3
  Flow Rate Source (TL)1/RConn1 -- DOWTHERM-A 2/LConn1

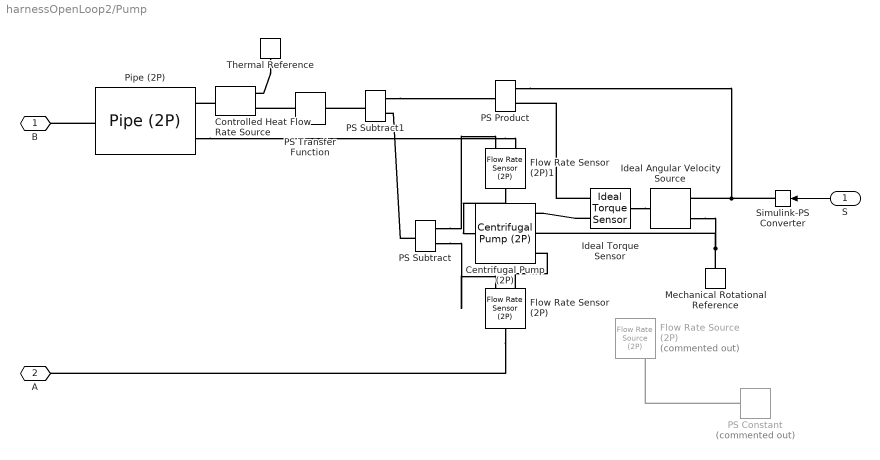
== system harnessOpenLoop2/Pump ==
  S : Inport
  Centrifugal Pump (2P) : SimscapeFluids_lib/Two-Phase Fluid/Fluid Machines/Centrifugal Pump (2P)  pump_parameterization=fluids.two_phase_fluid.fluid_machines.enum.CentrifugalPumpParameterization.Nominal  capacity_ref_nominal=Pump.nom_capacity lpm  head_ref_nominal=Pump.nom_head m  power_ref_nominal=Pump.nom_power kW  head_ref_max=Pump.max_head m  capacity_ref_max=Pump.max_capacity lpm  omega_ref_analytic=Pump.nom_speed rpm  capacity_ref_1D_TLU=[16.67, 30, 40, 53.33, 66.67, 83.33] lpm  head_ref_1D_TLU=[50, 47.5, 45, 40, 35, 25] m  power_ref_1D_TLU=[.6, .75, .85, .93, .98, .99] kW  omega_ref_1D=3500 rpm  rho_ref_1D=998.21 kg/m^3  omega_threshold_factor=1e-2  capacity_2D_TLU=[16.67, 23.33, 30, 40, 53.33, 60] lpm  omega_2D_TLU=[2450, 2800, 3150, 3500] rpm  head_2D_TLU=[25, 32.7, 42.5, 50; 24, 31.7, 41, 49; 22.7, 30.5, 39, 47.5; 20, 28, 36, 45; 15.7, 24, 32, 40; 12.5, 21, 29.5, 37.5] m  power_2D_TLU=[.28, .38, .5, .6; .31, .41, .55, .68; .33, .44, .6, .75; .36, .48, .65, .83; .38, .53, .72, .93; .39, .55, .75, .97] kW  rho_ref_2D=998.21 kg/m^3  diameter_ratio=1  mech_orientation=fluids.two_phase_fluid.fluid_machines.enum.CentrifugalPumpMechOrientation.Positive  area=0.01 m^2  liquid_check=simscape.enum.assert.action.warn  operation_check=simscape.enum.assert.action.none
      settings: InternalSimscapePortConfiguration="{\"Bottom\":[{\"id\":\"A\",\"label\":\"A\",\"type\":\"foundation.two_phase_fluid.two_phase_fluid\"}],\"Left\":[],\"Right\":[{\"id\":\"R\",\"label\":\"R\",\"type\":\"foundation.mechanical.rotational.rotational\"},{\"id\":\"C\",\"label\":\"C\",\"type\":\"foundation.mechanical.rotational.rotational\"}],\"Top\":[{\"id\":\"B\",\"label\":\"B\",\"type\":\"foundation.two_phase_fluid.two_phase_fluid\"}]}"
  Controlled Heat Flow Rate Source : fl_lib/Thermal/Thermal Sources/Controlled Heat Flow Rate Source
  Flow Rate Sensor (2P) : fl_lib/Two-Phase Fluid/Sensors/Flow Rate Sensor (2P)  mass_flow_measure=false  volumetric_flow_measure=false  energy_flow_measure=true
      settings: InternalSimscapePortConfiguration="{\"Bottom\":[{\"id\":\"PHI\",\"label\":\"φ\",\"type\":\"output\"}],\"Left\":[{\"id\":\"A\",\"label\":\"A\",\"type\":\"foundation.two_phase_fluid.two_phase_fluid\"}],\"Right\":[{\"id\":\"B\",\"label\":\"B\",\"type\":\"foundation.two_phase_fluid.two_phase_fluid\"}],\"Top\":[]}"
  Flow Rate Sensor (2P)1 : fl_lib/Two-Phase Fluid/Sensors/Flow Rate Sensor (2P)  mass_flow_measure=false  volumetric_flow_measure=false  energy_flow_measure=true
      settings: InternalSimscapePortConfiguration="{\"Bottom\":[{\"id\":\"PHI\",\"label\":\"φ\",\"type\":\"output\"}],\"Left\":[{\"id\":\"A\",\"label\":\"A\",\"type\":\"foundation.two_phase_fluid.two_phase_fluid\"}],\"Right\":[{\"id\":\"B\",\"label\":\"B\",\"type\":\"foundation.two_phase_fluid.two_phase_fluid\"}],\"Top\":[]}"
  Flow Rate Source (2P) : fl_lib/Two-Phase Fluid/Sources/Flow Rate Source (2P)  Commented=on  source_type=foundation.enum.constant_controlled.controlled  flow_type=foundation.enum.mass_volumetric_flow.mass  mass_flow=0 kg/s  volumetric_flow=0 m^3/s  power_spec=foundation.enum.power_spec.isentropic  area_A=0.01 m^2  area_B=0.01 m^2
      settings: InternalSimscapePortConfiguration="{\"Bottom\":[],\"Left\":[{\"id\":\"A\",\"label\":\"A\",\"type\":\"foundation.two_phase_fluid.two_phase_fluid\"},{\"id\":\"M\",\"label\":\"M\",\"type\":\"input\"}],\"Right\":[{\"id\":\"B\",\"label\":\"B\",\"type\":\"foundation.two_phase_fluid.two_phase_fluid\"}],\"Top\":[]}"
  Ideal Angular Velocity Source : fl_lib/Mechanical/Mechanical Sources/Ideal Angular Velocity Source
  Ideal Torque Sensor : fl_lib/Mechanical/Mechanical Sensors/Ideal Torque Sensor
  Mechanical Rotational Reference : fl_lib/Mechanical/Rotational Elements/Mechanical Rotational Reference
  PS Constant : fl_lib/Physical Signals/Sources/PS Constant  Commented=on  constant=NominalStates.mdot kg/s
  PS Product : fl_lib/Physical Signals/Functions/PS Product
  PS Subtract : fl_lib/Physical Signals/Functions/PS Subtract
  PS Subtract1 : fl_lib/Physical Signals/Functions/PS Subtract
  PS Transfer Function : fl_lib/Physical Signals/Linear Operators/PS Transfer Function  transfer_function_type=foundation.enum.transfer_function_type.lag  T=5 s  T1=2 s  T2=1 s  reset_method=foundation.enum.IntegratorResetSpec.None  initial_condition_spec=foundation.enum.IntegratorICSpec.Internal  y0=0 kW
      settings: InternalSimscapePortConfiguration="{\"Bottom\":[],\"Left\":[{\"id\":\"U\",\"label\":\"\",\"type\":\"input\"}],\"Right\":[{\"id\":\"Y\",\"label\":\"\",\"type\":\"output\"}],\"Top\":[]}"
  Pipe (2P) : fl_lib/Two-Phase Fluid/Elements/Pipe (2P)  length=0.5 m  area=0.01 m^2  Dh=0.1 m  length_add=0 m  roughness=15e-6 m  Re_lam=2000  Re_tur=4000  shape_factor=64  Nu_lam=3.66  inertia=false  energy_spec=foundation.enum.energy_spec.temperature  p_init=NominalStates.P(3) MPa  T_init=NominalStates.T(3) degC  x_init=0.5  alpha_init=0.5  h_init=1500 kJ/kg  u_init=1500 kJ/kg  mdot_init=0 kg/s  time_constant=0.1 s
      settings: InternalSimscapePortConfiguration="{\"Bottom\":[],\"Left\":[{\"id\":\"A\",\"label\":\"A\",\"type\":\"foundation.two_phase_fluid.two_phase_fluid\"},{\"id\":\"H\",\"label\":\"H\",\"type\":\"foundation.thermal.thermal\"}],\"Right\":[{\"id\":\"B\",\"label\":\"B\",\"type\":\"foundation.two_phase_fluid.two_phase_fluid\"}],\"Top\":[]}"
  Simulink-PS Converter : nesl_utility/Simulink-PS Converter  PhysicalDomain=network_engine_domain  SubClassName=ps_input  LeftPortType=input  RightPortType=output  PseudoPeriodic=off  Frequencies=[]  NoiseDistribution=none  NoiseParameters=[]  Unit=rpm  AffineConversion=off  FilteringAndDerivatives=provide  SimscapeFilterOrder=1  InputFilterTimeConstant=0.001  UdotUserProvided=0
  Thermal Reference : fl_lib/Thermal/Thermal Elements/Thermal Reference
  B : PMIOPort  Side=Left
  A : PMIOPort  Port=2  Side=Right
  wires:
  S/1 -> Simulink-PS Converter/1
  connections:
  Thermal Reference/LConn1 -- Controlled Heat Flow Rate Source/RConn2
  PS Subtract1/LConn1 -- PS Product/RConn1
  Simulink-PS Converter/RConn1 -- Ideal Angular Velocity Source/RConn1 -- PS Product/LConn1
  Flow Rate Sensor (2P)/RConn1 -- Centrifugal Pump (2P)/RConn3
  Flow Rate Sensor (2P)/LConn1 -- A/RConn1
  Ideal Torque Sensor/RConn2 -- PS Product/LConn2
  Ideal Torque Sensor/RConn1 -- Centrifugal Pump (2P)/RConn1
  PS Subtract1/RConn1 -- PS Transfer Function/LConn1
  Ideal Torque Sensor/LConn1 -- Ideal Angular Velocity Source/LConn1
  PS Subtract/LConn1 -- Flow Rate Sensor (2P)1/RConn2
  Mechanical Rotational Reference/LConn1 -- Centrifugal Pump (2P)/RConn2 -- Ideal Angular Velocity Source/RConn2
  PS Subtract/LConn2 -- Flow Rate Sensor (2P)/RConn2
  Pipe (2P)/RConn1 -- B/RConn1
  PS Transfer Function/RConn1 -- Controlled Heat Flow Rate Source/RConn1
  Controlled Heat Flow Rate Source/LConn1 -- Pipe (2P)/LConn2
  Pipe (2P)/LConn1 -- Flow Rate Sensor (2P)1/RConn1
  PS Subtract/RConn1 -- PS Subtract1/LConn2
  Flow Rate Sensor (2P)1/LConn1 -- Centrifugal Pump (2P)/LConn1
  PS Constant/RConn1 -- Flow Rate Source (2P)/LConn2

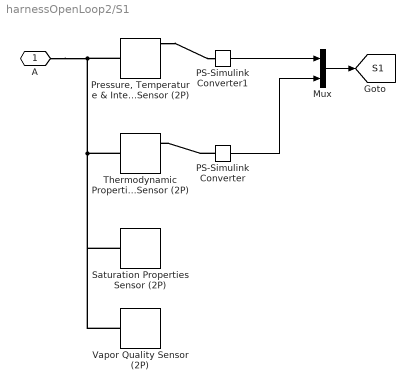
== system harnessOpenLoop2/S1 ==
  Mux : Mux  Inputs=2
  PS-Simulink Converter : nesl_utility/PS-Simulink Converter  PhysicalDomain=network_engine_domain  SubClassName=ps_output  LeftPortType=input  RightPortType=output  PseudoPeriodic=off  Frequencies=[]  VectorFormat=inherit  Unit=kJ/kg  AffineConversion=off
  PS-Simulink Converter1 : nesl_utility/PS-Simulink Converter  PhysicalDomain=network_engine_domain  SubClassName=ps_output  LeftPortType=input  RightPortType=output  PseudoPeriodic=off  Frequencies=[]  VectorFormat=inherit  Unit=MPa  AffineConversion=off
  "Pressure, Temperature & Internal Energy Sensor (2P)" : fl_lib/Two-Phase Fluid/Sensors/Pressure, Temperature & Internal Energy Sensor (2P)  reference=foundation.enum.MeasurementReference.absolute  pressure=true  pressure_spec=foundation.enum.PressureMeasementSpec.Absolute  temperature=true  internal_energy=true
      settings: InternalSimscapePortConfiguration="{\"Bottom\":[{\"id\":\"T\",\"label\":\"T\",\"type\":\"output\"},{\"id\":\"U\",\"label\":\"U\",\"type\":\"output\"}],\"Left\":[{\"id\":\"A\",\"label\":\"A\",\"type\":\"foundation.two_phase_fluid.two_phase_fluid\"}],\"Right\":[{\"id\":\"Pa\",\"label\":\"Pa\",\"type\":\"output\"}],\"Top\":[]}"
  Saturation Properties Sensor (2P) : fl_lib/Two-Phase Fluid/Sensors/Saturation Properties Sensor (2P)  temperature_measure=true  pressure_measure=false  pressure_check=simscape.enum.assert.action.error  energy_measure=foundation.enum.EnergyMeasurement.Off  density_measure=foundation.enum.DensityMeasurement.Off
      settings: InternalSimscapePortConfiguration="{\"Bottom\":[],\"Left\":[{\"id\":\"A\",\"label\":\"A\",\"type\":\"foundation.two_phase_fluid.two_phase_fluid\"}],\"Right\":[{\"id\":\"T_sat_liq\",\"label\":\"TL\",\"type\":\"output\"},{\"id\":\"T_sat_vap\",\"label\":\"TV\",\"type\":\"output\"}],\"Top\":[]}"
  Thermodynamic Properties Sensor (2P) : fl_lib/Two-Phase Fluid/Sensors/Thermodynamic Properties Sensor (2P)  temperature=true  enthalpy=true  density=true  specific_volume=true  entropy=true
      settings: InternalSimscapePortConfiguration="{\"Bottom\":[{\"id\":\"V\",\"label\":\"v\",\"type\":\"output\"},{\"id\":\"S\",\"label\":\"s\",\"type\":\"output\"}],\"Left\":[{\"id\":\"A\",\"label\":\"A\",\"type\":\"foundation.two_phase_fluid.two_phase_fluid\"}],\"Right\":[{\"id\":\"T\",\"label\":\"T\",\"type\":\"output\"},{\"id\":\"H\",\"label\":\"h\",\"type\":\"output\"},{\"id\":\"RHO\",\"label\":\"ρ\",\"type\":\"output\"}],\"Top\":[]}"
  Vapor Quality Sensor (2P) : fl_lib/Two-Phase Fluid/Sensors/Vapor Quality Sensor (2P)  vapor_fraction_spec=foundation.enum.vapor_fraction_spec.quality
      settings: InternalSimscapePortConfiguration="{\"Bottom\":[],\"Left\":[{\"id\":\"A\",\"label\":\"A\",\"type\":\"foundation.two_phase_fluid.two_phase_fluid\"}],\"Right\":[{\"id\":\"X\",\"label\":\"X\",\"type\":\"output\"}],\"Top\":[]}"
  A : PMIOPort  Side=Left
  tag scope: S1=global
  wires:
  PS-Simulink Converter/1 -> Mux/2
  PS-Simulink Converter1/1 -> Mux/1
  Mux/1 -> [S1]
  connections:
  Thermodynamic Properties Sensor (2P)/LConn1 -- Vapor Quality Sensor (2P)/LConn1 -- Saturation Properties Sensor (2P)/LConn1 -- A/RConn1 -- "Pressure, Temperature & Internal Energy Sensor (2P)"/LConn1
  PS-Simulink Converter/LConn1 -- Thermodynamic Properties Sensor (2P)/RConn2
  "Pressure, Temperature & Internal Energy Sensor (2P)"/RConn1 -- PS-Simulink Converter1/LConn1

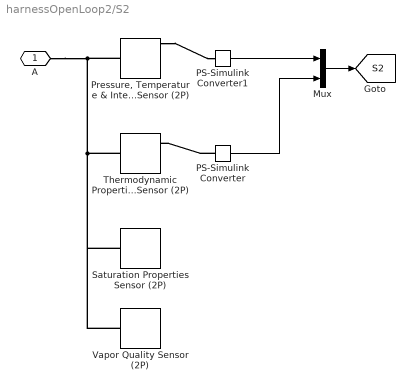
== system harnessOpenLoop2/S2 ==
  Mux : Mux  Inputs=2
  PS-Simulink Converter : nesl_utility/PS-Simulink Converter  PhysicalDomain=network_engine_domain  SubClassName=ps_output  LeftPortType=input  RightPortType=output  PseudoPeriodic=off  Frequencies=[]  VectorFormat=inherit  Unit=kJ/kg  AffineConversion=off
  PS-Simulink Converter1 : nesl_utility/PS-Simulink Converter  PhysicalDomain=network_engine_domain  SubClassName=ps_output  LeftPortType=input  RightPortType=output  PseudoPeriodic=off  Frequencies=[]  VectorFormat=inherit  Unit=MPa  AffineConversion=off
  "Pressure, Temperature & Internal Energy Sensor (2P)" : fl_lib/Two-Phase Fluid/Sensors/Pressure, Temperature & Internal Energy Sensor (2P)  reference=foundation.enum.MeasurementReference.absolute  pressure=true  pressure_spec=foundation.enum.PressureMeasementSpec.Absolute  temperature=true  internal_energy=true
      settings: InternalSimscapePortConfiguration="{\"Bottom\":[{\"id\":\"T\",\"label\":\"T\",\"type\":\"output\"},{\"id\":\"U\",\"label\":\"U\",\"type\":\"output\"}],\"Left\":[{\"id\":\"A\",\"label\":\"A\",\"type\":\"foundation.two_phase_fluid.two_phase_fluid\"}],\"Right\":[{\"id\":\"Pa\",\"label\":\"Pa\",\"type\":\"output\"}],\"Top\":[]}"
  Saturation Properties Sensor (2P) : fl_lib/Two-Phase Fluid/Sensors/Saturation Properties Sensor (2P)  temperature_measure=true  pressure_measure=false  pressure_check=simscape.enum.assert.action.error  energy_measure=foundation.enum.EnergyMeasurement.Off  density_measure=foundation.enum.DensityMeasurement.Off
      settings: InternalSimscapePortConfiguration="{\"Bottom\":[],\"Left\":[{\"id\":\"A\",\"label\":\"A\",\"type\":\"foundation.two_phase_fluid.two_phase_fluid\"}],\"Right\":[{\"id\":\"T_sat_liq\",\"label\":\"TL\",\"type\":\"output\"},{\"id\":\"T_sat_vap\",\"label\":\"TV\",\"type\":\"output\"}],\"Top\":[]}"
  Thermodynamic Properties Sensor (2P) : fl_lib/Two-Phase Fluid/Sensors/Thermodynamic Properties Sensor (2P)  temperature=true  enthalpy=true  density=true  specific_volume=true  entropy=true
      settings: InternalSimscapePortConfiguration="{\"Bottom\":[{\"id\":\"V\",\"label\":\"v\",\"type\":\"output\"},{\"id\":\"S\",\"label\":\"s\",\"type\":\"output\"}],\"Left\":[{\"id\":\"A\",\"label\":\"A\",\"type\":\"foundation.two_phase_fluid.two_phase_fluid\"}],\"Right\":[{\"id\":\"T\",\"label\":\"T\",\"type\":\"output\"},{\"id\":\"H\",\"label\":\"h\",\"type\":\"output\"},{\"id\":\"RHO\",\"label\":\"ρ\",\"type\":\"output\"}],\"Top\":[]}"
  Vapor Quality Sensor (2P) : fl_lib/Two-Phase Fluid/Sensors/Vapor Quality Sensor (2P)  vapor_fraction_spec=foundation.enum.vapor_fraction_spec.quality
      settings: InternalSimscapePortConfiguration="{\"Bottom\":[],\"Left\":[{\"id\":\"A\",\"label\":\"A\",\"type\":\"foundation.two_phase_fluid.two_phase_fluid\"}],\"Right\":[{\"id\":\"X\",\"label\":\"X\",\"type\":\"output\"}],\"Top\":[]}"
  A : PMIOPort  Side=Left
  tag scope: S2=global
  wires:
  Mux/1 -> [S2]
  PS-Simulink Converter1/1 -> Mux/1
  PS-Simulink Converter/1 -> Mux/2
  connections:
  "Pressure, Temperature & Internal Energy Sensor (2P)"/RConn1 -- PS-Simulink Converter1/LConn1
  PS-Simulink Converter/LConn1 -- Thermodynamic Properties Sensor (2P)/RConn2
  Saturation Properties Sensor (2P)/LConn1 -- Vapor Quality Sensor (2P)/LConn1 -- Thermodynamic Properties Sensor (2P)/LConn1 -- "Pressure, Temperature & Internal Energy Sensor (2P)"/LConn1 -- A/RConn1

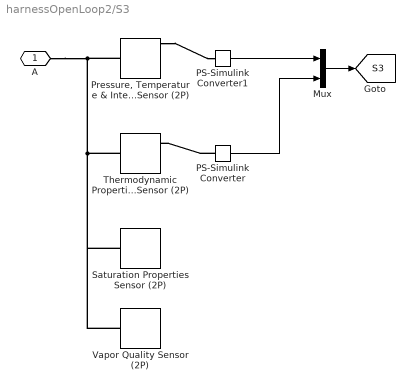
== system harnessOpenLoop2/S3 ==
  Mux : Mux  Inputs=2
  PS-Simulink Converter : nesl_utility/PS-Simulink Converter  PhysicalDomain=network_engine_domain  SubClassName=ps_output  LeftPortType=input  RightPortType=output  PseudoPeriodic=off  Frequencies=[]  VectorFormat=inherit  Unit=kJ/kg  AffineConversion=off
  PS-Simulink Converter1 : nesl_utility/PS-Simulink Converter  PhysicalDomain=network_engine_domain  SubClassName=ps_output  LeftPortType=input  RightPortType=output  PseudoPeriodic=off  Frequencies=[]  VectorFormat=inherit  Unit=MPa  AffineConversion=off
  "Pressure, Temperature & Internal Energy Sensor (2P)" : fl_lib/Two-Phase Fluid/Sensors/Pressure, Temperature & Internal Energy Sensor (2P)  reference=foundation.enum.MeasurementReference.absolute  pressure=true  pressure_spec=foundation.enum.PressureMeasementSpec.Absolute  temperature=true  internal_energy=true
      settings: InternalSimscapePortConfiguration="{\"Bottom\":[{\"id\":\"T\",\"label\":\"T\",\"type\":\"output\"},{\"id\":\"U\",\"label\":\"U\",\"type\":\"output\"}],\"Left\":[{\"id\":\"A\",\"label\":\"A\",\"type\":\"foundation.two_phase_fluid.two_phase_fluid\"}],\"Right\":[{\"id\":\"Pa\",\"label\":\"Pa\",\"type\":\"output\"}],\"Top\":[]}"
  Saturation Properties Sensor (2P) : fl_lib/Two-Phase Fluid/Sensors/Saturation Properties Sensor (2P)  temperature_measure=true  pressure_measure=false  pressure_check=simscape.enum.assert.action.error  energy_measure=foundation.enum.EnergyMeasurement.Off  density_measure=foundation.enum.DensityMeasurement.Off
      settings: InternalSimscapePortConfiguration="{\"Bottom\":[],\"Left\":[{\"id\":\"A\",\"label\":\"A\",\"type\":\"foundation.two_phase_fluid.two_phase_fluid\"}],\"Right\":[{\"id\":\"T_sat_liq\",\"label\":\"TL\",\"type\":\"output\"},{\"id\":\"T_sat_vap\",\"label\":\"TV\",\"type\":\"output\"}],\"Top\":[]}"
  Thermodynamic Properties Sensor (2P) : fl_lib/Two-Phase Fluid/Sensors/Thermodynamic Properties Sensor (2P)  temperature=true  enthalpy=true  density=true  specific_volume=true  entropy=true
      settings: InternalSimscapePortConfiguration="{\"Bottom\":[{\"id\":\"V\",\"label\":\"v\",\"type\":\"output\"},{\"id\":\"S\",\"label\":\"s\",\"type\":\"output\"}],\"Left\":[{\"id\":\"A\",\"label\":\"A\",\"type\":\"foundation.two_phase_fluid.two_phase_fluid\"}],\"Right\":[{\"id\":\"T\",\"label\":\"T\",\"type\":\"output\"},{\"id\":\"H\",\"label\":\"h\",\"type\":\"output\"},{\"id\":\"RHO\",\"label\":\"ρ\",\"type\":\"output\"}],\"Top\":[]}"
  Vapor Quality Sensor (2P) : fl_lib/Two-Phase Fluid/Sensors/Vapor Quality Sensor (2P)  vapor_fraction_spec=foundation.enum.vapor_fraction_spec.quality
      settings: InternalSimscapePortConfiguration="{\"Bottom\":[],\"Left\":[{\"id\":\"A\",\"label\":\"A\",\"type\":\"foundation.two_phase_fluid.two_phase_fluid\"}],\"Right\":[{\"id\":\"X\",\"label\":\"X\",\"type\":\"output\"}],\"Top\":[]}"
  A : PMIOPort  Side=Left
  tag scope: S3=global
  wires:
  PS-Simulink Converter/1 -> Mux/2
  PS-Simulink Converter1/1 -> Mux/1
  Mux/1 -> [S3]
  connections:
  A/RConn1 -- "Pressure, Temperature & Internal Energy Sensor (2P)"/LConn1 -- Thermodynamic Properties Sensor (2P)/LConn1 -- Vapor Quality Sensor (2P)/LConn1 -- Saturation Properties Sensor (2P)/LConn1
  PS-Simulink Converter/LConn1 -- Thermodynamic Properties Sensor (2P)/RConn2
  "Pressure, Temperature & Internal Energy Sensor (2P)"/RConn1 -- PS-Simulink Converter1/LConn1
